simulink model "Model_H3_Ase_Gusts_Pid"  (Simulink 6.3)
settings: Solver=ode45  StartTime=tmin  StopTime=tmax  MaxStep=dt  RelTol=1e-3  AbsTol=1e-6
values from neighbouring files (symbols this model uses):
  dt = 0.01    [Pgm_G11_Superposition.m]    (also in Pgm_G12_Num_Integration.m; Pgm_G13_Frequency_Domain.m = 0.0625; Pgm_H2_Response_Gusts_Control.m = 0.001; Pgm_H3_Ase_Gusts_Pid.m = 0.001)
  MC = inv(A)*C    [Pgm_H2_Response_Gusts_Control.m]    (also in Pgm_H3_Ase_Gusts_Pid.m; Pgm_I6_Dynamic_Manoeuvres.m = inv(M) * C; Pgm_I7_Gust_Time.m = MI * CC; Pgm_I91_Taxiing.m = inv(M) * CC)
  MFG = inv(A)*F_gust    [Pgm_H2_Response_Gusts_Control.m]    (also in Pgm_H3_Ase_Gusts_Pid.m)
  MK = inv(A)*K    [Pgm_H2_Response_Gusts_Control.m]    (also in Pgm_H3_Ase_Gusts_Pid.m; Pgm_I7_Gust_Time.m = MI * KK; Pgm_I91_Taxiing.m = inv(M) * K)
settings Model: LastModifiedBy=jecooper  StrictBusMsg=None
settings DataIOCC: SignalLoggingName=sigsOut
settings DebuggingCC: SolverPrmCheckMsg=none
settings HardwareCC: TargetUnknown=on
settings GRTTargetCC: ModelReferenceCompliant=off  MatFileLogging=off

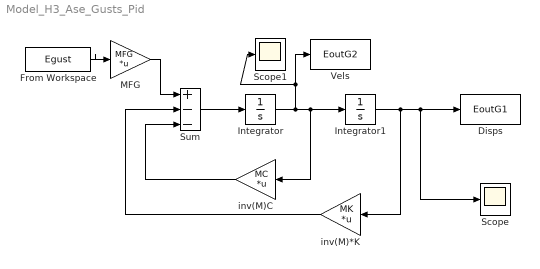
== system Model_H3_Ase_Gusts_Pid ==
  Disps : ToWorkspace  VariableName=EoutG1  SampleTime=dt  SaveFormat=Array
  From Workspace : FromWorkspace  VariableName=Egust  SampleTime=dt
  Integrator : Integrator
  Integrator1 : Integrator
  MFG : Gain  Gain=MFG  Multiplication=Matrix(K*u) (u vector)  SaturateOnIntegerOverflow=on
  Scope : Scope
      settings: YMin=-1.25  YMax=1.25
  Scope1 : Scope
      settings: YMin=-80  YMax=80
  Sum : Sum  Inputs=+--  SaturateOnIntegerOverflow=on
  Vels : ToWorkspace  VariableName=EoutG2  SampleTime=dt  SaveFormat=Array
  inv(M)*K : Gain  Orientation=left  Gain=MK  Multiplication=Matrix(K*u)  SaturateOnIntegerOverflow=on
  inv(M)C : Gain  Orientation=left  Gain=MC  Multiplication=Matrix(K*u)  SaturateOnIntegerOverflow=on
  wires:
  Integrator/1 -> Integrator1/1, inv(M)C/1, Vels/1, Scope1/1
  Sum/1 -> Integrator/1
  Integrator1/1 -> Disps/1, Scope/1, inv(M)*K/1
  From Workspace/1 -> MFG/1
  MFG/1 -> Sum/1
  inv(M)C/1 -> Sum/3
  inv(M)*K/1 -> Sum/2
